simulink model "Audio_Display"  (R2021a)
settings: Solver=VariableStepAuto  StartTime=0.0  StopTime=inf  RelTol=1e-3
libraries: dspfdesign x2, dspsnks4 x1, dspvision x1, dspindex x1
settings Model: Creator=arthur  LastModifiedBy=arthur

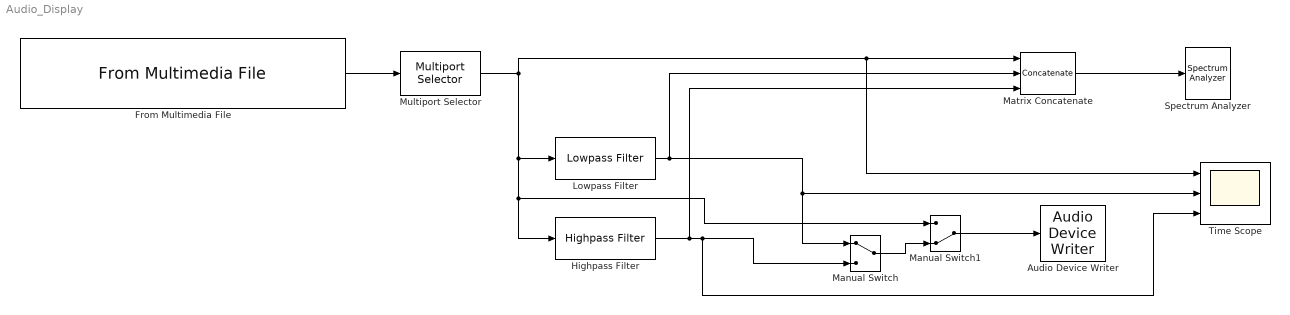
== system Audio_Display ==
  Audio Device Writer : dspsnks4/Audio Device Writer  Driver=CoreAudio  Device=Haut-parleurs MacBook Air  InheritSampleRate=on  SampleRate=44100  BitDepth=16-bit integer  BufferSize=4096  NumBuffers=10  DefaultOutputChannelMapping=on  OutputChannelMapping=1:2  OutputNumUnderrunSamples=off  DriverIdx=5  DeviceWarnFlag=''
  From Multimedia File : dspvision/From Multimedia File  inputFilename=/Users/arthur/Documents/Documents - MacBook Air de Arthur/GitHub/dut_rt/RTAM2107/PAPACITO_BA_EXPEDITION_PUNITIVE.mp3  readRange=[1 Inf]  loop=on  numPlays=inf  outputStreams=Audio only  videoDataType=single  audioDataType=double  inheritSampleTime=on  userDefinedSampleTime=1/30  noAudioOutput=off  isIntensityVideo=off  fourcc=RGB  colorVideoFormat=Separate color signals  outputEOF=off  dataOrg=Column-major  audioFrameSize=124  computeAudioFrameSize=off  outSamplingMode=Sample based
  Highpass Filter : dspfdesign/Highpass Filter  FilterType=FIR  DesignForMinimumOrder=on  FilterOrder=50  StopbandFrequency=3e3  PassbandFrequency=4e3  StopbandAttenuation=80  PassbandRipple=0.1  InheritSampleRate=off  SampleRate=44100  SimulateUsing=Interpreted execution  roundingMode=Floor  coeffsDataTypeStr=fixdt(1,16)
  Lowpass Filter : dspfdesign/Lowpass Filter  FilterType=FIR  DesignForMinimumOrder=on  FilterOrder=50  PassbandFrequency=3e3  StopbandFrequency=4e3  PassbandRipple=0.1  StopbandAttenuation=80  InheritSampleRate=off  SampleRate=44100  SimulateUsing=Interpreted execution  roundingMode=Floor  coeffsDataTypeStr=fixdt(1,16)
  Manual Switch : ManualSwitch
  Manual Switch1 : ManualSwitch  CurrentSetting=0
  Matrix Concatenate : Concatenate  NumInputs=3  Mode=Multidimensional array  ConcatenateDimension=2
  Multiport Selector : dspindex/Multiport Selector  rowsOrCols=Columns  idxCellArray={1}  idxErrMode=Clip Index
  Spectrum Analyzer : SpectrumAnalyzer
  Time Scope : Scope  NumInputPorts=3
  wires:
  From Multimedia File/1 -> Multiport Selector/1
  Multiport Selector/1 -> Time Scope/1, Matrix Concatenate/1, Highpass Filter/1, Manual Switch1/1, Lowpass Filter/1
  Highpass Filter/1 -> Matrix Concatenate/3, Time Scope/3, Manual Switch/2
  Lowpass Filter/1 -> Matrix Concatenate/2, Manual Switch/1, Time Scope/2
  Manual Switch/1 -> Manual Switch1/2
  Manual Switch1/1 -> Audio Device Writer/1
  Matrix Concatenate/1 -> Spectrum Analyzer/1
